simulink model "narmamaglev"  (Simulink 8.8)
settings: Solver=ode45  StartTime=0.0  StopTime=30  RelTol=1e-3  AbsTol=1e-6
undefined symbols (not defined in the file): now, sfunxy2
settings Model: Creator=The MathWorks, Inc.  LastModifiedBy=The MathWorks, Inc.  ExtModeTrigMode=oneshot  ExtModeArmWhenConnect=off  TunableVars=prueba  TunableVarsStorageClass=Auto
settings DataIOCC: LimitDataPoints=off  SignalLoggingSaveFormat=Dataset  SaveOutput=off  SignalLoggingName=sigsOut
settings OptimizationCC: BooleanDataType=off  DefaultParameterBehavior=Inlined  ExpressionDepthLimit=2147483647  InitFltsAndDblsToZero=on
settings DebuggingCC: SaveWithParameterizedLinksMsg=none  SignalResolutionControl=TryResolveAllWithWarning  MultiTaskDSMMsg=warning  MultiTaskCondExecSysMsg=none  StrictBusMsg=None
settings HardwareCC: TargetUnknown=on
settings RTWCC: TemplateMakefile=grt_vc.tmf
settings GRTTargetCC: TargetFcnLib=ansi_tfl_tmw.mat

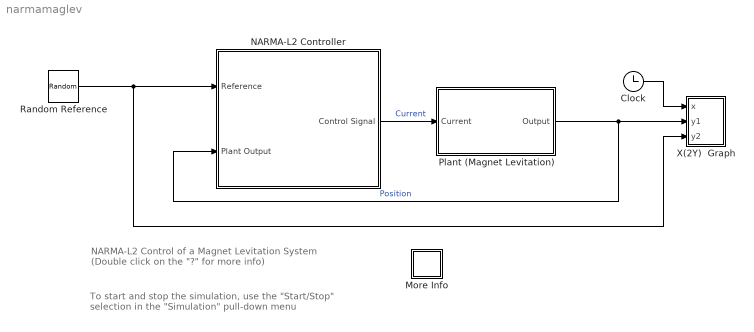
== system narmamaglev ==
  note: NARMA-L2 Control of a Magnet Levitation System
      | (Double click on the "?" for more info)
  note: To start and stop the simulation, use the "Start/Stop"
      | selection in the "Simulation" pull-down menu
  Clock : Clock
  More Info : Subsystem
      mask Display: disp('?')
  NARMA-L2 Controller : Subsystem  mask(NARMA-L2 Controller){Ts=0.01, S1=9, Ni=3, Nj=2, sim_file=ballrepel0, trainfun=trainlm, Use_validation=1, Use_Testing=1, max_i=4, min_i=-1, max_i_int=1, min_i_int=0.1, sam_training=10000, epochs=100, minp=-0.98589809892637514, maxp=3.9504698574991721, mint=-0.0016503994509919615, maxt=5.8483552223055346, Normalize=1, IW1_1=[2.8589406503354526 3.8571763260787164 2.4456184377322217 0.8666607644547214;0.84908220491155217 -0.74479667271080674 0.17438611819566038 -0.054598878873029347;-0.62709936825321444 -1.3691145688669635 -1.0354349321363878 -2.2482593652050578;-0.61112872012274111 3.6328637614421511 -2.9819224741551729 3.7430014139229799;8.2151216183173048 -0.34864518388745791 -0.63898245756720395 3.2213765524683398;-0.62348046801820789 1.6654556537092802 -0.62194271006861923 0.21912328150625099;0.14622178875562497 0.092672072012439946 -2.0000544306046777 -1.7404534095664805;-0.016488785105071693 0.16978381724998215 -0.084822329865259866 0.026867941830282197;1.9174811964991516 -1.6949195923894798 0.35217636039029204 -0.12168945961699514], IW3_2=[2.0947814145837365 4.1399235297823935 0.45973664424051686 1.4201813933844121;-0.86879079197788289 -0.91114493693130993 -1.7736957440317072 -1.8251383343645129;-1.5220230282736409 -1.9645557493380605 -0.13454356275803814 0.69198422228505774;1.1049207565072356 1.1058960542907463 -1.644921307204396 -0.10202375847256849;1.762641725993455 0.12377706028660714 -0.7437018195796895 1.3293490471370206;1.390274388145605 1.2487181342609894 0.59892762333675664 1.8687582044711111;-1.2477149308688809 -0.79236132307758722 0.36202987325836317 -2.3538403428029064;-1.795434452809733 0.33077476751858431 1.195152886823688 -0.75536654530187719;1.5958944923973373 -0.67233970442189994 2.0385698345589716 1.2983707063666041], IW5_3=-0.86130222828051506, LW2_1=[0.00015172623864271055 2.2013108252986395 -0.00041943793424466811 -0.0003479657571070474 -4.886121844237561e-005 0.048716164660783372 0.00018521862399574861 4.7909859890519924 0.47215204119265081], LW4_3=[1.1881559217746376 1.4377070715786655 -0.90278040876764909 -2.3370997753198059 -0.097223533841072435 -0.63741922080667701 -2.7337228147947257 3.0132329690414466 2.17298689321732], LW5_4=0.599679883882549, LW6_5=0.00053164383570330738, LW6_2=1.015263173451765, B1=[-2.0509205219588469;-0.31031398693333401;-1.4045705779285507;0.015391387074643211;-3.2845781323270051;1.1180253626502208;2.2612148765562523;-0.13759375641734173;1.1010317884774456], B2=0.89897272661230299, B3=[-1.002095836800059;-1.126799288887316;1.0075534076876089;3.6052646447174865;-0.024716746631406297;1.2795222700572257;-2.288460695586839;-3.073994760224549;1.7909749466641665], B4=0.8642380934413868, Limit_output=1, min_output=0, max_output=Inf, Use_Previous_Weights=1}
      mask prompts: Ts "Sample time"; trainfun "Training function"
      mask help: NARMA-L2 Controller. You first train a neural network model of the plant to be controlled. The controller is a rearrangement of the trained plant model. Double-click the NARMA-L2 Controller block to begin the plant training.
      mask init:
      | xl = [0    .4   NaN  .33  .55   .55  .33  .33  NaN .80  .92 .92];
      | yl = [.95 .95 NaN  .75  .75   .55  .55  .75  NaN  .95 .95 .65];
      | x2 = [0    .43 NaN .45 .45    NaN .92 1.2 NaN .63 .85 .85 .63 .63 ];
      | y2 = [.39 .39 NaN  .41 .55   NaN .65 .65 NaN .75 .75  .55  .55  .75];
      | x3 = [.45 .45 NaN .42 .45 .48  NaN .33 .4 .33];
      | y3 = [.75 .90 NaN .83 .90 .83  NaN  .98 .95 .92];
      | x4 = [.75 .75 NaN .72 .75 .78  NaN  .5 .7 NaN .63 .7 .63];
      | y4 = [.75 .90 NaN .83 .90 .83  NaN .95 .95 NaN .98 .95 .92];
      | x5 = [.43 .43 .77 .77 .43 NaN .36 .43 .36 NaN .75 .75];
      | y5 = [.37 .41 .41 .37 .37 NaN .42 .39 .36 NaN .41 .55];
      | x6 = [.92 .92 .77 NaN .84 .77 .84];
      | y6 = [.65 .39 .39 NaN .42 .39 .36];
      | x1t=.03; y1t=.31;
      | x2t=.03; y2t=.85;
      | x8t=.03;y8t=.21;
      | x3t=.77; y3t=.53;
      | x4t=.77; y4t=.44;
      | x5t=.34; y5t=.49;
      | x6t=.58; y6t=.49;
      | 
      | 
      | t=(0:24)/24*2*pi;
      | xs = .05*cos(t);
      | ys = .05*sin(t);
      | xs1=xs+.45;
      | ys1=ys+.95;
      | xs2=xs+.75;
      | ys2=ys+.95;
      settings: OpenFcn=nncontrolutil('nnident','',gcbh,gcb,'narma_l2');
      mask TypeOptions trainfun: trainbfg | trainbr  | traincgb | traincgf | traincgp | traingd | traingdm | traingda | traingdx | trainlm  | trainoss | trainrp  | trainscg
      mask Display:
      | plot([[xl NaN x2]*.9-.075 ], [[yl  NaN y2]*.9-.1 ]);
      | plot([[x3 NaN xs1 NaN xs2]*.9-.075 ], [[y3 NaN ys1 NaN ys2]*.9-.1 ]);
      | plot([x4 NaN x5]*.9-.075,[y4 NaN y5]*.9-.1);
      | plot([x6 NaN ]*.9-.075,[y6 NaN ]*.9-.1);
      | text(x1t,y1t,'Plant');
      | text(x8t,y8t,'Output');
      | text(x2t,y2t,'Reference');
      | text(x3t,y3t,'Control');
      | text(x4t,y4t,'Signal');
      | text(x5t,y5t,'f');
      | text(x6t,y6t,'g');
  Plant (Magnet Levitation) : Subsystem
      mask init:
      | x1=[-2 -2 2 2 -2 NaN -2 -2 2 2 -2];
      | y1=[5 4 4 5 5 NaN 2 0 0 2 2];
      | x2=[-2 -2 2 2 -2 NaN -2   2  NaN -2 2 NaN 2    4    NaN 2  4];
      | y2=[4  3  3 4  4 NaN 1.5 1  NaN 1 .5 NaN 1.5 1.5 NaN .5 .5];
      | x1t = -.5 ; y1t = 4.4;
      | x2t = -.5; y2t = 3.4;
      mask Display:
      | plot([-10],[0],[10],[5]);
      | plot([x1 NaN x2],[y1 NaN y2]);
      | text(x1t,y1t,'N')
      | text(x2t,y2t,'S')
  Random Reference : UniformRandomNumber  Minimum=0.5  Maximum=4  Seed=round(now)  SampleTime=5
  X(2Y)  Graph : Subsystem  LoadFcn=sfunxy2([],[],[],'LoadBlock')  StartFcn=sfunxy2([],[],[],'Start')  StopFcn=sfunxy2([],[],[],'Stop')  mask(X(2Y) scope.){xmin=0, xmax=5, ymin=-1, ymax=1, st=-1}
      mask prompts: xmin "x-min:"; xmax "x-max:"; ymin "y-min:"; ymax "y-max:"; st "Sample time:"
      mask help: X(2Y) scope using MATLAB graph window. First input is used as time base. Enter plotting ranges.
      settings: CopyFcn=sfunxy2([],[],[],'CopyBlock')  DeleteFcn=sfunxy2([],[],[],'DeleteBlock')  NameChangeFcn=sfunxy2([],[],[],'NameChange')
      mask Help: This block can be used to explore limit cycles. Look at the function sfunxy.m to see how it works.
      mask Display: plot([.05 .95 .95 .05 .05],[.45 .45 .95 .95 .45], 0.5+cos(0:0.1:2*pi)*0.3,0.7+sin(0:0.1:2*pi)*0.2)
  wires:
  Clock/1 -> X(2Y)  Graph/1(x)
  Random Reference/1 -> X(2Y)  Graph/3(y2), NARMA-L2 Controller/1(Reference)
  NARMA-L2 Controller/1(Control Signal) -> Plant (Magnet Levitation)/1(Current)  "Current"
  Plant (Magnet Levitation)/1(Output) -> NARMA-L2 Controller/2(Plant Output), X(2Y)  Graph/2(y1)  "Position"

== system narmamaglev/More Info ==
  note: This system simulates NARMA-L2 control
      | of a magnet suspended by an electromagnet.
  note: Double-click on the NARMA-L2 Controller block
      | to train the neural network controller and plant model.
  note: For more information on what the controller
      | does, look under the mask of the NARMA-L2
      | Controller block.

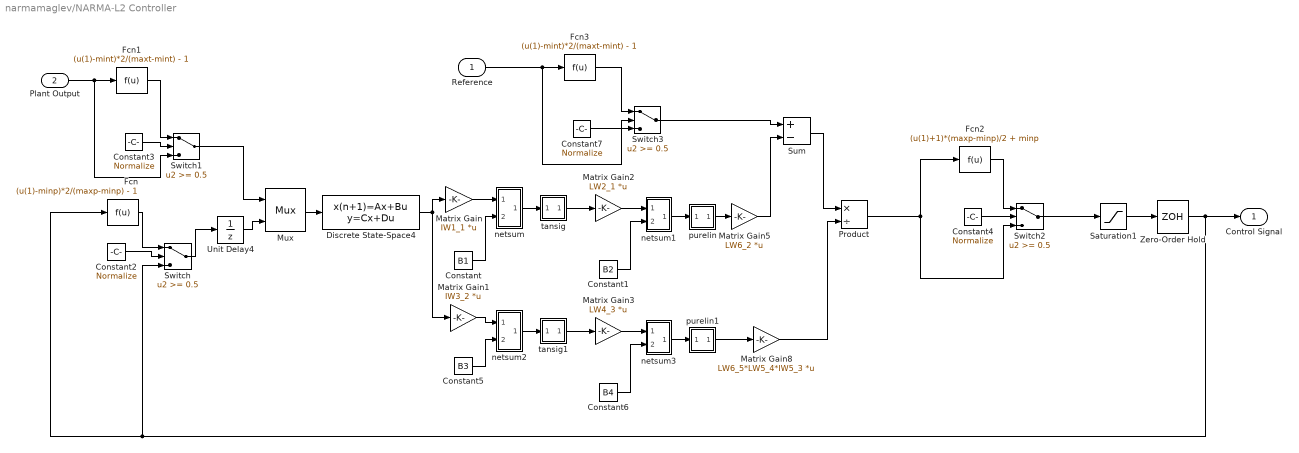
== system narmamaglev/NARMA-L2 Controller ==
  Reference : Inport
  Plant Output : Inport  Port=2
  Constant : Constant  Value=B1
  Constant1 : Constant  Value=B2
  Constant{2..4,7} (4 alike) : Constant  Value=Normalize
  Constant5 : Constant  Value=B3
  Constant6 : Constant  Value=B4
  Discrete State-Space4 : DiscreteStateSpace  A=blkdiag([zeros(1,Nj-1);eye(Nj-2,Nj-2) zeros(Nj-2,1)],[zeros(1,Ni-1);eye(Ni-2,Ni-2) zeros(Ni-2,1)])  B=blkdiag(eye(Nj-1,1),eye(Ni-1,1))  C=blkdiag([zeros(1,Nj-1);eye(Nj-1,Nj-1)],[zeros(eye(double(Ni>1)),Ni-1);eye(Ni-2,Ni-1)])  D=blkdiag([1;zeros(Nj-1,1)],[eye(double(Ni>1));zeros(Ni-2,1)])  SampleTime=Ts
  Fcn : Fcn  Expr=(u(1)-minp)*2/(maxp-minp) - 1
  Fcn1 : Fcn  Expr=(u(1)-mint)*2/(maxt-mint) - 1
  Fcn2 : Fcn  Expr=(u(1)+1)*(maxp-minp)/2 + minp
  Fcn3 : Fcn  Expr=(u(1)-mint)*2/(maxt-mint) - 1
  Matrix Gain : Gain  Gain=IW1_1  Multiplication=Matrix(K*u)  SaturateOnIntegerOverflow=on  OutDataTypeStr=Inherit: Same as input  ParamDataTypeStr=Inherit: Same as input
  Matrix Gain1 : Gain  Gain=IW3_2  Multiplication=Matrix(K*u)  SaturateOnIntegerOverflow=on  OutDataTypeStr=Inherit: Same as input  ParamDataTypeStr=Inherit: Same as input
  Matrix Gain2 : Gain  Gain=LW2_1  Multiplication=Matrix(K*u)  SaturateOnIntegerOverflow=on  OutDataTypeStr=Inherit: Same as input  ParamDataTypeStr=Inherit: Same as input
  Matrix Gain3 : Gain  Gain=LW4_3  Multiplication=Matrix(K*u)  SaturateOnIntegerOverflow=on  OutDataTypeStr=Inherit: Same as input  ParamDataTypeStr=Inherit: Same as input
  Matrix Gain5 : Gain  Gain=LW6_2  Multiplication=Matrix(K*u)  SaturateOnIntegerOverflow=on  OutDataTypeStr=Inherit: Same as input  ParamDataTypeStr=Inherit: Same as input
  Matrix Gain8 : Gain  Gain=LW6_5*LW5_4*IW5_3  Multiplication=Matrix(K*u)  SaturateOnIntegerOverflow=on  OutDataTypeStr=Inherit: Same as input  ParamDataTypeStr=Inherit: Same as input
  Mux : Mux  Inputs=2
      settings: DisplayOption=signals
  Product : Product  Inputs=*/  SaturateOnIntegerOverflow=on  InputSameDT=on  OutDataTypeStr=Inherit: Same as first input
  Saturation1 : Saturate  UpperLimit=max_i  LowerLimit=min_i  ZeroCross=off
  Sum : Sum  Inputs=+-  SaturateOnIntegerOverflow=on  InputSameDT=on  OutDataTypeStr=Inherit: Same as first input
  Switch{,1..3} (4 alike) : Switch  Threshold=0.5  ZeroCross=off  SaturateOnIntegerOverflow=on  InputSameDT=on
  Unit Delay4 : UnitDelay  SampleTime=Ts
  Zero-Order Hold : ZeroOrderHold  SampleTime=Ts
  netsum : Subsystem
      mask Display: disp('+')
  netsum1 : Subsystem
      mask Display: disp('+')
  netsum2 : Subsystem
      mask Display: disp('+')
  netsum3 : Subsystem
      mask Display: disp('+')
  purelin : Subsystem
      mask Display: plot([-1 1],[0 0],[-1 1],[-1 1])
  purelin1 : Subsystem
      mask Display: plot([-1 1],[0 0],[-1 1],[-1 1])
  tansig : Subsystem
      mask Display: plot([-1 1],[0 0],[-1 -.9 -.8 -.7 -.6 -.5 -.4 -.3 -.2 -.1 0 .1 .2 .3 .4 .5 .6 .7 .8 .9 1],2./(1+exp(-8*[-1 -.9 -.8 -.7 -.6 -.5 -.4 -.3 -.2 -.1 0 .1 .2 .3 .4 .5 .6 .7 .8 .9 1]))-1)
  tansig1 : Subsystem
      mask Display: plot([-1 1],[0 0],[-1 -.9 -.8 -.7 -.6 -.5 -.4 -.3 -.2 -.1 0 .1 .2 .3 .4 .5 .6 .7 .8 .9 1],2./(1+exp(-8*[-1 -.9 -.8 -.7 -.6 -.5 -.4 -.3 -.2 -.1 0 .1 .2 .3 .4 .5 .6 .7 .8 .9 1]))-1)
  Control Signal : Outport
  wires:
  Constant3/1 -> Switch1/2
  Fcn1/1 -> Switch1/1
  Plant Output/1 -> Fcn1/1, Switch1/3
  netsum1/1(Out1) -> purelin/1(n)
  Constant1/1 -> netsum1/2(In2)
  Matrix Gain2/1 -> netsum1/1(In1)
  netsum/1(Out1) -> tansig/1(n)
  Constant/1 -> netsum/2(In2)
  tansig/1(a) -> Matrix Gain2/1
  Matrix Gain/1 -> netsum/1(In1)
  netsum3/1(Out1) -> purelin1/1(n)
  Constant6/1 -> netsum3/2(In2)
  Matrix Gain3/1 -> netsum3/1(In1)
  netsum2/1(Out1) -> tansig1/1(n)
  Constant5/1 -> netsum2/2(In2)
  tansig1/1(a) -> Matrix Gain3/1
  Matrix Gain1/1 -> netsum2/1(In1)
  purelin/1(a) -> Matrix Gain5/1
  Matrix Gain5/1 -> Sum/2
  Sum/1 -> Product/1
  purelin1/1(a) -> Matrix Gain8/1
  Matrix Gain8/1 -> Product/2
  Constant7/1 -> Switch3/2
  Fcn3/1 -> Switch3/1
  Reference/1 -> Fcn3/1, Switch3/3
  Switch3/1 -> Sum/1
  Switch1/1 -> Mux/1
  Mux/1 -> Discrete State-Space4/1
  Discrete State-Space4/1 -> Matrix Gain/1, Matrix Gain1/1
  Zero-Order Hold/1 -> Control Signal/1, Fcn/1, Switch/3
  Fcn/1 -> Switch/1
  Constant2/1 -> Switch/2
  Unit Delay4/1 -> Mux/2
  Switch/1 -> Unit Delay4/1
  Saturation1/1 -> Zero-Order Hold/1
  Product/1 -> Fcn2/1, Switch2/3
  Constant4/1 -> Switch2/2
  Switch2/1 -> Saturation1/1
  Fcn2/1 -> Switch2/1

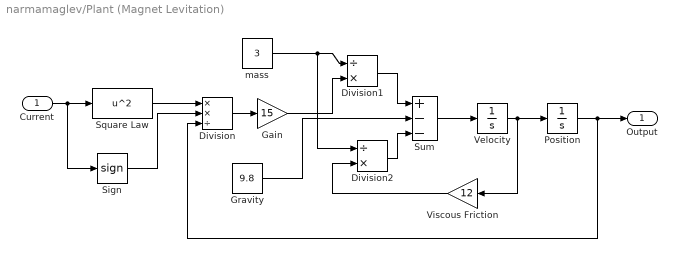
== system narmamaglev/Plant (Magnet Levitation) ==
  Current : Inport
  Division : Product  Inputs=**/  SaturateOnIntegerOverflow=on  InputSameDT=on  OutDataTypeStr=Inherit: Same as first input
  Division1 : Product  Inputs=/*  SaturateOnIntegerOverflow=on  InputSameDT=on  OutDataTypeStr=Inherit: Same as first input
  Division2 : Product  Inputs=/*  SaturateOnIntegerOverflow=on  InputSameDT=on  OutDataTypeStr=Inherit: Same as first input
  Gain : Gain  Gain=15  SaturateOnIntegerOverflow=on  OutDataTypeStr=Inherit: Same as input  ParamDataTypeStr=Inherit: Same as input
  Gravity : Constant  Value=9.8
  Position : Integrator  InitialCondition=.5  ZeroCross=off
  Sign : Signum  ZeroCross=off
  Square Law : Fcn  Expr=u^2
  Sum : Sum  Inputs=|+--  SaturateOnIntegerOverflow=on  InputSameDT=on  OutDataTypeStr=Inherit: Same as first input
  Velocity : Integrator  ZeroCross=off
  Viscous Friction : Gain  Gain=12  SaturateOnIntegerOverflow=on  OutDataTypeStr=Inherit: Same as input  ParamDataTypeStr=Inherit: Same as input
  mass : Constant  Value=3
  Output : Outport
  wires:
  Square Law/1 -> Division/1
  Division/1 -> Gain/1
  Gravity/1 -> Sum/2
  Velocity/1 -> Position/1, Viscous Friction/1
  Sum/1 -> Velocity/1
  Gain/1 -> Division1/2
  Division1/1 -> Sum/1
  mass/1 -> Division1/1, Division2/1
  Viscous Friction/1 -> Division2/2
  Division2/1 -> Sum/3
  Current/1 -> Square Law/1, Sign/1
  Position/1 -> Output/1, Division/3
  Sign/1 -> Division/2

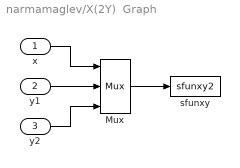
== system narmamaglev/X(2Y)  Graph ==
  x : Inport
  y1 : Inport  Port=2
  y2 : Inport  Port=3
  Mux : Mux  Inputs=3
  sfunxy : S-Function  FunctionName=sfunxy2  Parameters=[xmin xmax ymin ymax], st  SFunctionDeploymentMode=off  EnableBusSupport=off
  wires:
  y2/1 -> Mux/3
  y1/1 -> Mux/2
  x/1 -> Mux/1
  Mux/1 -> sfunxy/1

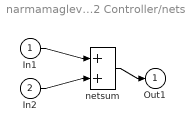
== system narmamaglev/NARMA-L2 Controller/netsum ==
  In1 : Inport
  In2 : Inport  Port=2
  netsum : Sum  Inputs=2  SaturateOnIntegerOverflow=on  InputSameDT=on  OutDataTypeStr=Inherit: Same as first input
  Out1 : Outport
  wires:
  In1/1 -> netsum/1
  In2/1 -> netsum/2
  netsum/1 -> Out1/1

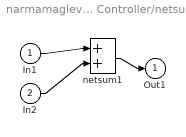
== system narmamaglev/NARMA-L2 Controller/netsum1 ==
  In1 : Inport
  In2 : Inport  Port=2
  netsum1 : Sum  Inputs=2  SaturateOnIntegerOverflow=on  InputSameDT=on  OutDataTypeStr=Inherit: Same as first input
  Out1 : Outport
  wires:
  In1/1 -> netsum1/1
  In2/1 -> netsum1/2
  netsum1/1 -> Out1/1

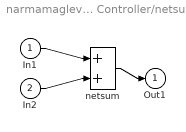
== system narmamaglev/NARMA-L2 Controller/netsum2 ==
  In1 : Inport
  In2 : Inport  Port=2
  netsum : Sum  Inputs=2  SaturateOnIntegerOverflow=on  InputSameDT=on  OutDataTypeStr=Inherit: Same as first input
  Out1 : Outport
  wires:
  In1/1 -> netsum/1
  In2/1 -> netsum/2
  netsum/1 -> Out1/1

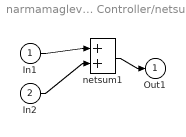
== system narmamaglev/NARMA-L2 Controller/netsum3 ==
  In1 : Inport
  In2 : Inport  Port=2
  netsum1 : Sum  Inputs=2  SaturateOnIntegerOverflow=on  InputSameDT=on  OutDataTypeStr=Inherit: Same as first input
  Out1 : Outport
  wires:
  In1/1 -> netsum1/1
  In2/1 -> netsum1/2
  netsum1/1 -> Out1/1

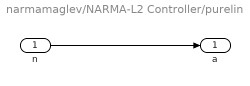
== system narmamaglev/NARMA-L2 Controller/purelin ==
  n : Inport
  a : Outport
  wires:
  n/1 -> a/1

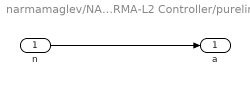
== system narmamaglev/NARMA-L2 Controller/purelin1 ==
  n : Inport
  a : Outport
  wires:
  n/1 -> a/1

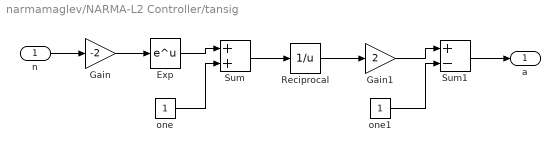
== system narmamaglev/NARMA-L2 Controller/tansig ==
  n : Inport
  Exp : Math  SaturateOnIntegerOverflow=on
  Gain : Gain  Gain=-2  SaturateOnIntegerOverflow=on  OutDataTypeStr=Inherit: Same as input  ParamDataTypeStr=Inherit: Same as input
  Gain1 : Gain  Gain=2  SaturateOnIntegerOverflow=on  OutDataTypeStr=Inherit: Same as input  ParamDataTypeStr=Inherit: Same as input
  Reciprocal : Math  Operator=reciprocal  SaturateOnIntegerOverflow=on
  Sum : Sum  SaturateOnIntegerOverflow=on  InputSameDT=on  OutDataTypeStr=Inherit: Same as first input
  Sum1 : Sum  Inputs=+-  SaturateOnIntegerOverflow=on  InputSameDT=on  OutDataTypeStr=Inherit: Same as first input
  one : Constant
  one1 : Constant
  a : Outport
  wires:
  n/1 -> Gain/1
  Gain/1 -> Exp/1
  Exp/1 -> Sum/1
  one/1 -> Sum/2
  Sum/1 -> Reciprocal/1
  Reciprocal/1 -> Gain1/1
  Gain1/1 -> Sum1/1
  one1/1 -> Sum1/2
  Sum1/1 -> a/1

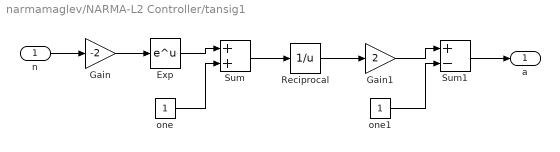
== system narmamaglev/NARMA-L2 Controller/tansig1 ==
  n : Inport
  Exp : Math  SaturateOnIntegerOverflow=on
  Gain : Gain  Gain=-2  SaturateOnIntegerOverflow=on  OutDataTypeStr=Inherit: Same as input  ParamDataTypeStr=Inherit: Same as input
  Gain1 : Gain  Gain=2  SaturateOnIntegerOverflow=on  OutDataTypeStr=Inherit: Same as input  ParamDataTypeStr=Inherit: Same as input
  Reciprocal : Math  Operator=reciprocal  SaturateOnIntegerOverflow=on
  Sum : Sum  SaturateOnIntegerOverflow=on  InputSameDT=on  OutDataTypeStr=Inherit: Same as first input
  Sum1 : Sum  Inputs=+-  SaturateOnIntegerOverflow=on  InputSameDT=on  OutDataTypeStr=Inherit: Same as first input
  one : Constant
  one1 : Constant
  a : Outport
  wires:
  n/1 -> Gain/1
  Gain/1 -> Exp/1
  Exp/1 -> Sum/1
  one/1 -> Sum/2
  Sum/1 -> Reciprocal/1
  Reciprocal/1 -> Gain1/1
  Gain1/1 -> Sum1/1
  one1/1 -> Sum1/2
  Sum1/1 -> a/1
